simulink model "Task4_4"  (R2020b)
settings: Solver=ode23t  StartTime=0.0  StopTime=300  FixedStep=1e-4  RelTol=1e-3
values from neighbouring files (symbols this model uses):
  Cp_opt = lambda_opt * Ct_opt    (= 0.4375971)    [Code2021_Jo_Saleh.m]    (also in ExeRet21.m.m)
  Ct = c0 + c1.*lambda + c2*lambda.^2    [Code2021_Jo_Saleh.m]    (also in ExeRet21.m.m)
  i_sd_mat = zeros(1, length(Te))    [Code2021_Jo_Saleh.m]    (also in ExeRet21.m.m)
  i_sq_mat = zeros(1, length(Te))    [Code2021_Jo_Saleh.m]    (also in ExeRet21.m.m)
  J = H * 2 * Sb / wm^2    (= 9574851.8542)    [Code2021_Jo_Saleh.m]    (also in ExeRet21.m.m)
  K = p * tau_z / (tau_pl * 2*we * tau_w)    (= -13.4008504823)    [Code2021_Jo_Saleh.m]    (also in ExeRet21.m.m)
  Kd_i = Rs * Kd_p / Lsd    (= -20)    [Code2021_Jo_Saleh.m]    (also in ExeRet21.m.m)
  Kd_p = - Lsd / tau_i    (= -2)    [Code2021_Jo_Saleh.m]    (also in ExeRet21.m.m)
  Kq_i = Rs * Kq_p / Lsq    (= -20)    [Code2021_Jo_Saleh.m]    (also in ExeRet21.m.m)
  Kq_p = - Lsq / tau_i    (= -2.66666666667)    [Code2021_Jo_Saleh.m]    (also in ExeRet21.m.m)
  lambda_opt = 6.7    [Code2021_Jo_Saleh.m]    (also in ExeRet21.m.m)
  Lsd = 6e-3    (= 0.006)    [Code2021_Jo_Saleh.m]    (also in ExeRet21.m.m)
  Lsq = 8e-3    (= 0.008)    [Code2021_Jo_Saleh.m]    (also in ExeRet21.m.m)
  p = 180    [Code2021_Jo_Saleh.m]    (also in ExeRet21.m.m)
  Phi_m = 17.3    [Code2021_Jo_Saleh.m]    (also in ExeRet21.m.m)
  r = 50    [Code2021_Jo_Saleh.m]    (also in ExeRet21.m.m)
  rho = 1.225    [Code2021_Jo_Saleh.m]    (also in ExeRet21.m.m)
  Rs = 60e-3    (= 0.06)    [Code2021_Jo_Saleh.m]    (also in ExeRet21.m.m)
  tau_le = tau_w    (= 8.82652066845)    [Code2021_Jo_Saleh.m]    (also in ExeRet21.m.m)
  tau_lg = tau_z    (= -109.330180381)    [Code2021_Jo_Saleh.m]    (also in ExeRet21.m.m)
  Te = 0:1e3:Te_rated    [Code2021_Jo_Saleh.m]    (also in ExeRet21.m.m)
  Te_rated = (Ptur * p) / (2 * we)    (= 1671126.90246)    [Code2021_Jo_Saleh.m]    (also in ExeRet21.m.m)
  Vdc = 6e3    (= 6000)    [Code2021_Jo_Saleh.m]    (also in ExeRet21.m.m)
libraries: pid_lib x2
settings Model: Creator=Tomo  LastModifiedBy=Tomo

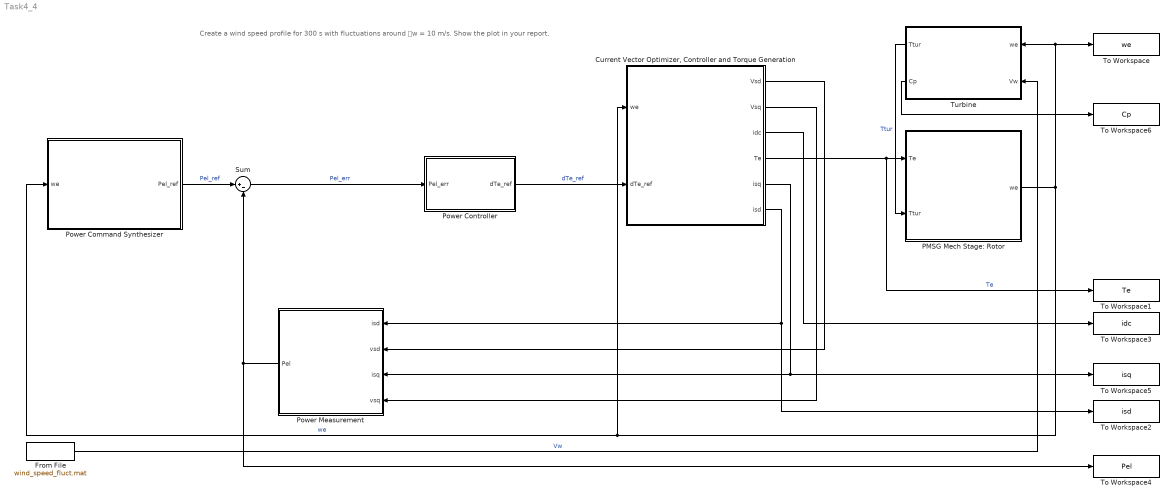
== system Task4_4 ==
  note: Create a wind speed profile for 300 s with fluctuations around 𝑉w = 10 m/s. Show the plot in your report.
  "Current Vector Optimizer, Controller and Torque Generation" : Subsystem
  From File : FromFile  FileName=wind_speed_fluct.mat  SampleTime=0
  PMSG Mech Stage: Rotor : Subsystem
  Power Command Synthesizer : Subsystem
  Power Controller : Subsystem
  Power Measurement : Subsystem
  Sum : Sum  Inputs=|+-
  To Workspace : ToWorkspace  VariableName=we  SampleTime=-1
  To Workspace1 : ToWorkspace  VariableName=Te  SampleTime=-1
  To Workspace2 : ToWorkspace  VariableName=isd  SampleTime=-1
  To Workspace3 : ToWorkspace  VariableName=idc  SampleTime=-1
  To Workspace4 : ToWorkspace  VariableName=Pel  SampleTime=-1
  To Workspace5 : ToWorkspace  VariableName=isq  SampleTime=-1
  To Workspace6 : ToWorkspace  VariableName=Cp  SampleTime=-1
  Turbine : Subsystem
  wires:
  "Current Vector Optimizer, Controller and Torque Generation"/3(idc) -> To Workspace3/1
  "Current Vector Optimizer, Controller and Torque Generation"/4(Te) -> To Workspace1/1, PMSG Mech Stage: Rotor/1(Te)  "Te"
  Power Measurement/1(Pel) -> Sum/2, To Workspace4/1
  "Current Vector Optimizer, Controller and Torque Generation"/2(Vsq) -> Power Measurement/4(vsq)
  Sum/1 -> Power Controller/1(Pel_err)  "Pel_err"
  From File/1 -> Turbine/2(Vw)  "Vw"
  PMSG Mech Stage: Rotor/1(we) -> "Current Vector Optimizer, Controller and Torque Generation"/1(we), Power Command Synthesizer/1(we), To Workspace/1, Turbine/1(we)  "we"
  "Current Vector Optimizer, Controller and Torque Generation"/6(isd) -> To Workspace2/1, Power Measurement/1(isd)
  Turbine/1(Ttur) -> PMSG Mech Stage: Rotor/2(Ttur)  "Ttur"
  Power Command Synthesizer/1(Pel_ref) -> Sum/1  "Pel_ref"
  "Current Vector Optimizer, Controller and Torque Generation"/5(isq) -> To Workspace5/1, Power Measurement/3(isq)
  Power Controller/1(dTe_ref) -> "Current Vector Optimizer, Controller and Torque Generation"/2(dTe_ref)  "dTe_ref"
  "Current Vector Optimizer, Controller and Torque Generation"/1(Vsd) -> Power Measurement/2(vsd)
  Turbine/2(Cp) -> To Workspace6/1

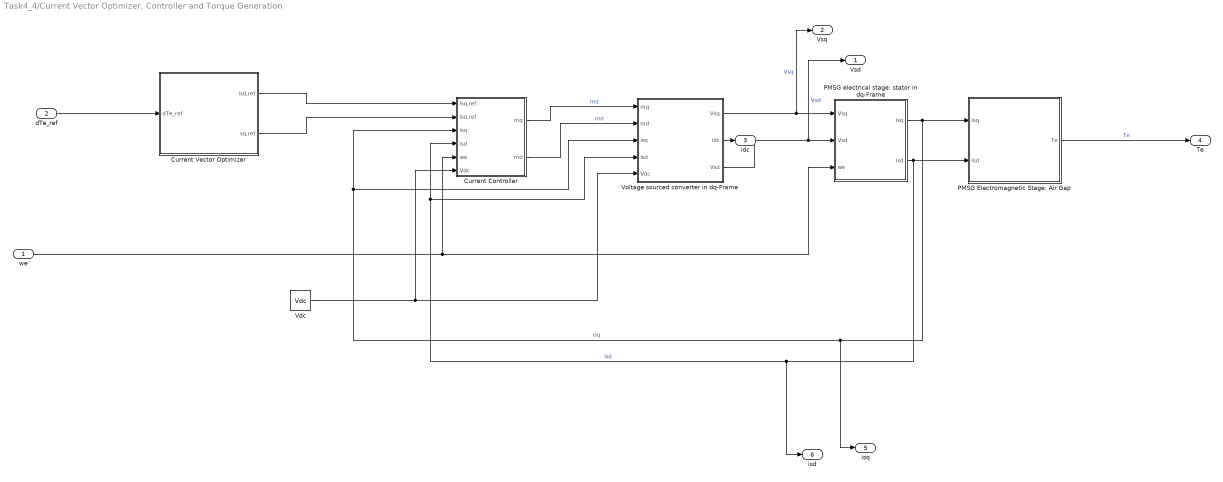
== system Task4_4/Current Vector Optimizer, Controller and Torque Generation ==
  we : Inport
  dTe_ref : Inport  Port=2
  Current Controller : Subsystem
  Current Vector Optimizer : Subsystem
  PMSG Electromagnetic Stage: Air Gap : Subsystem
  PMSG electrical stage: stator in dq-Frame : Subsystem
  Vdc : Constant  Value=Vdc
  Voltage sourced converter in dq-Frame : Subsystem
  Vsd : Outport
  Vsq : Outport  Port=2
  idc : Outport  Port=3
  Te : Outport  Port=4
  isq : Outport  Port=5
  isd : Outport  Port=6
  wires:
  PMSG electrical stage: stator in dq-Frame/1(isq) -> isq/1, Voltage sourced converter in dq-Frame/3(isq), Current Controller/3(isq), PMSG Electromagnetic Stage: Air Gap/1(Isq)  "isq"
  PMSG Electromagnetic Stage: Air Gap/1(Te) -> Te/1  "Te"
  Vdc/1 -> Voltage sourced converter in dq-Frame/5(Vdc), Current Controller/6(Vdc)
  Current Controller/2(md) -> Voltage sourced converter in dq-Frame/2(md)  "md"
  Current Controller/1(mq) -> Voltage sourced converter in dq-Frame/1(mq)  "mq"
  Voltage sourced converter in dq-Frame/1(Vsq) -> Vsq/1, PMSG electrical stage: stator in dq-Frame/1(Vsq)  "Vsq"
  Current Vector Optimizer/2(sq,ref) -> Current Controller/2(isd,ref)
  we/1 -> PMSG electrical stage: stator in dq-Frame/3(we), Current Controller/5(we)
  Voltage sourced converter in dq-Frame/3(Vsd) -> Vsd/1, PMSG electrical stage: stator in dq-Frame/2(Vsd)  "Vsd"
  PMSG electrical stage: stator in dq-Frame/2(isd) -> PMSG Electromagnetic Stage: Air Gap/2(Isd), isd/1, Voltage sourced converter in dq-Frame/4(isd), Current Controller/4(isd)  "isd"
  Current Vector Optimizer/1(isd,ref) -> Current Controller/1(isq,ref)
  Voltage sourced converter in dq-Frame/2(idc) -> idc/1
  dTe_ref/1 -> Current Vector Optimizer/1(dTe_ref)

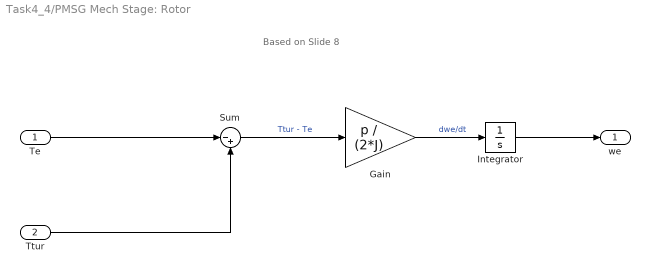
== system Task4_4/PMSG Mech Stage: Rotor ==
  note: Based on Slide 8
  Te : Inport
  Ttur : Inport  Port=2
  Gain : Gain  Gain=p / (2*J)
  Integrator : Integrator  InitialCondition=10
  Sum : Sum  Inputs=|-+
  we : Outport
  wires:
  Gain/1 -> Integrator/1  "dwe/dt"
  Integrator/1 -> we/1
  Sum/1 -> Gain/1  "Ttur - Te"
  Te/1 -> Sum/1
  Ttur/1 -> Sum/2

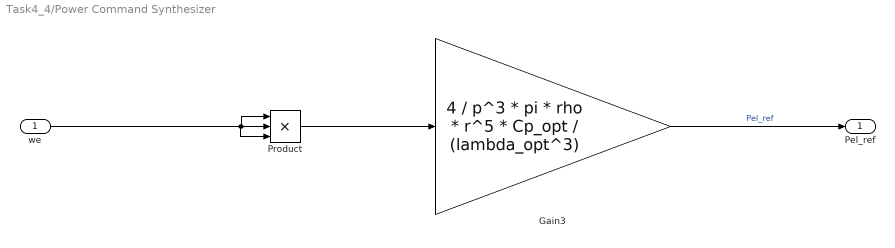
== system Task4_4/Power Command Synthesizer ==
  we : Inport
  Gain3 : Gain  Gain=4 / p^3 * pi * rho * r^5 * Cp_opt / (lambda_opt^3)
  Product : Product  Inputs=3
  Pel_ref : Outport
  wires:
  we/1 -> Product/2, Product/1, Product/3
  Gain3/1 -> Pel_ref/1  "Pel_ref"
  Product/1 -> Gain3/1

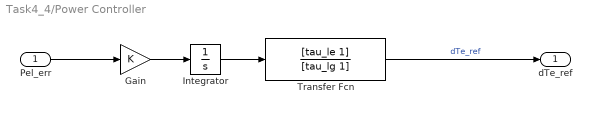
== system Task4_4/Power Controller ==
  Pel_err : Inport
  Gain : Gain  Gain=K
  Integrator : Integrator  InitialCondition=Te_rated
  Transfer Fcn : TransferFcn  Numerator=[tau_le 1]  Denominator=[tau_lg 1]
  dTe_ref : Outport
  wires:
  Transfer Fcn/1 -> dTe_ref/1  "dTe_ref"
  Gain/1 -> Integrator/1
  Integrator/1 -> Transfer Fcn/1
  Pel_err/1 -> Gain/1

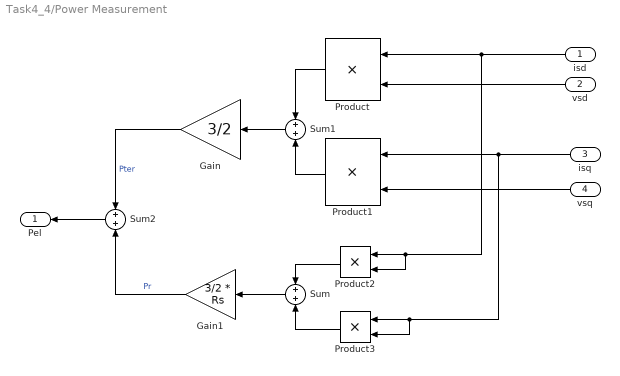
== system Task4_4/Power Measurement ==
  isd : Inport
  vsd : Inport  Port=2
  isq : Inport  Port=3
  vsq : Inport  Port=4
  Gain : Gain  Gain=3/2
  Gain1 : Gain  Gain=3/2 * Rs
  Product{,1..3} (4 alike) : Product
  Sum : Sum  Inputs=+|+
  Sum1 : Sum  Inputs=+|+
  Sum2 : Sum  Inputs=+|+
  Pel : Outport
  wires:
  Product/1 -> Sum1/1
  Sum1/1 -> Gain/1
  vsd/1 -> Product/2
  vsq/1 -> Product1/2
  Gain/1 -> Sum2/1  "Pter"
  isd/1 -> Product2/2, Product2/1, Product/1
  Product1/1 -> Sum1/2
  isq/1 -> Product3/2, Product3/1, Product1/1
  Sum/1 -> Gain1/1
  Product2/1 -> Sum/1
  Product3/1 -> Sum/2
  Gain1/1 -> Sum2/2  "Pr"
  Sum2/1 -> Pel/1

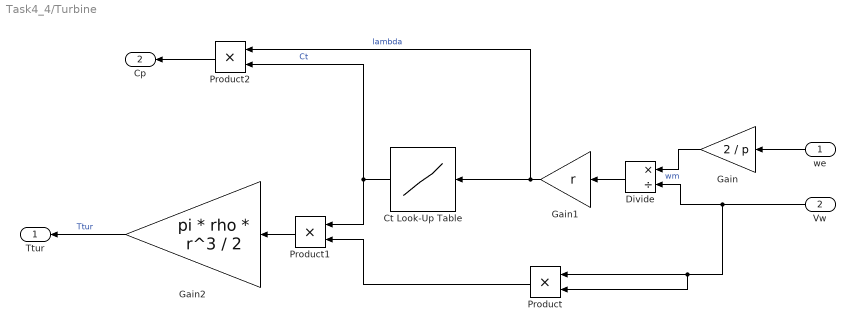
== system Task4_4/Turbine ==
  we : Inport
  Vw : Inport  Port=2
  Ct Look-Up Table : Lookup_n-D  NumberOfTableDimensions=1  BreakpointsForDimension1=[0:1e-2:20]  Table=Ct  InternalRulePriority=Speed  RndMeth=Simplest  InputSameDT=on
  Divide : Product  Inputs=*/
  Gain : Gain  Gain=2 / p
  Gain1 : Gain  Gain=r
  Gain2 : Gain  Gain=pi * rho * r^3 / 2
  Product : Product
  Product1 : Product
  Product2 : Product
  Ttur : Outport
  Cp : Outport  Port=2
  wires:
  we/1 -> Gain/1
  Gain2/1 -> Ttur/1  "Ttur"
  Ct Look-Up Table/1 -> Product1/1, Product2/2  "Ct"
  Gain/1 -> Divide/1  "wm"
  Gain1/1 -> Product2/1, Ct Look-Up Table/1  "lambda"
  Vw/1 -> Product/2, Product/1, Divide/2
  Divide/1 -> Gain1/1
  Product/1 -> Product1/2
  Product1/1 -> Gain2/1
  Product2/1 -> Cp/1

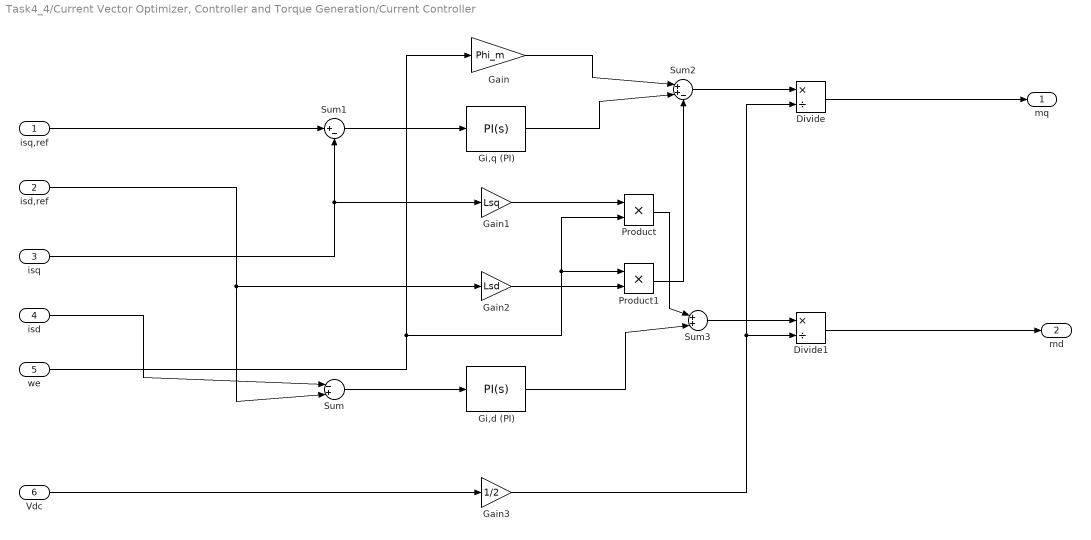
== system Task4_4/Current Vector Optimizer, Controller and Torque Generation/Current Controller ==
  isq,ref : Inport
  isd,ref : Inport  Port=2
  isq : Inport  Port=3
  isd : Inport  Port=4
  we : Inport  Port=5
  Vdc : Inport  Port=6
  Divide : Product  Inputs=*/
  Divide1 : Product  Inputs=*/
  Gain : Gain  Gain=Phi_m
  Gain1 : Gain  Gain=Lsq
  Gain2 : Gain  Gain=Lsd
  Gain3 : Gain  Gain=1/2
  Gi,d (PI) : pid_lib/PID Controller  Controller=PI  Form=Parallel  TimeDomain=Continuous-time  UseExternalTs=off  SampleTime=-1  IntegratorMethod=Forward Euler  FilterMethod=Forward Euler  ControllerParametersSource=internal  P=Kd_p  I=Kd_i  D=0  UseFilter=on  N=100  TunerSelectOption=Transfer Function Based (PID Tuner App)  InitialConditionSource=internal  InitialConditionForIntegrator=0  InitialConditionForFilter=0  DifferentiatorICPrevScaledInput=0  ExternalReset=none  TrackingMode=off  Kt=1  LimitOutput=off  SatLimitsSource=internal  UpperSaturationLimit=inf  LowerSaturationLimit=-inf  LinearizeAsGain=on  AntiWindupMode=none  Kb=1  POutMin=[]  POutMax=[]  IOutMin=[]  IOutMax=[]  DOutMin=[]  DOutMax=[]  NOutMin=[]  NOutMax=[]  SumOutMin=[]  SumOutMax=[]  SaturationOutMin=[]  SaturationOutMax=[]  PParamMin=[]  PParamMax=[]  IParamMin=[]  IParamMax=[]  DParamMin=[]  DParamMax=[]  NParamMin=[]  NParamMax=[]  KbParamMin=[]  KbParamMax=[]  KtParamMin=[]  KtParamMax=[]  KbOutMin=[]  KbOutMax=[]  KtOutMin=[]  KtOutMax=[]  IntegratorOutMin=[]  IntegratorOutMax=[]  FilterOutMin=[]  FilterOutMax=[]  SumI1OutMin=[]  SumI1OutMax=[]  SumI2OutMin=[]  SumI2OutMax=[]  SumI3OutMin=[]  SumI3OutMax=[]  SumI4OutMin=[]  SumI4OutMax=[]  SumDOutMin=[]  SumDOutMax=[]  DifferentiatorOutMin=[]  DifferentiatorOutMax=[]  FilterDiffOutCoefMin=[]  FilterDiffOutCoefMax=[]  ReciprocalOutMin=[]  ReciprocalOutMax=[]  SumDenOutMin=[]  SumDenOutMax=[]  SumNumOutMin=[]  SumNumOutMax=[]  DivideOutMin=[]  DivideOutMax=[]  UdiffTsProdOutMin=[]  UdiffTsProdOutMax=[]  NTsProdOutMin=[]  NTsProdOutMax=[]  UintegralTsProdOutMin=[]  UintegralTsProdOutMax=[]  UngainTsProdOutMin=[]  UngainTsProdOutMax=[]  IntegratorContinuousStateAttributes=''  IntegratorStateMustResolveToSignalObject=off  IntegratorRTWStateStorageClass=Auto  FilterContinuousStateAttributes=''  FilterStateMustResolveToSignalObject=off  FilterRTWStateStorageClass=Auto  ParallelPVariant=InternalParameters  IdealPVariant=Disabled  IVariant=InternalParameters  DVariant=Disabled  IntegratorVariant=Continuous  SatVariant=Disabled  AWVariant=Passthrough  PCopyVariant=Disabled  TRVariant=Disabled  FdbkBlocksVariant=Forward  IdealPFdbkVariant=Disabled  SatFdbkVariant=Disabled  DerivativeFilterVariant=Disabled  NVariant=Disabled  NCopyVariant=Disabled_SignalSpec  FilterICVariant=Disabled  IntegratorICVariant=InternalICs  ExternalResetVariant=Disabled  TRSumVariant=Passthrough  SumFdbkVariant=Disabled  SumVariant=Sum_PI  TsampFilterVariant=InternalTs  TsampNgainVariant=Passthrough  TsampIntegralVariant=Passthrough  ExternalSaturationOutDataTypeStr=Inherit: Same as second input
  Gi,q (PI) : pid_lib/PID Controller  Controller=PI  Form=Parallel  TimeDomain=Continuous-time  UseExternalTs=off  SampleTime=-1  IntegratorMethod=Forward Euler  FilterMethod=Forward Euler  ControllerParametersSource=internal  P=Kq_p  I=Kq_i  D=0  UseFilter=on  N=100  TunerSelectOption=Transfer Function Based (PID Tuner App)  InitialConditionSource=internal  InitialConditionForIntegrator=0  InitialConditionForFilter=0  DifferentiatorICPrevScaledInput=0  ExternalReset=none  TrackingMode=off  Kt=1  LimitOutput=off  SatLimitsSource=internal  UpperSaturationLimit=inf  LowerSaturationLimit=-inf  LinearizeAsGain=on  AntiWindupMode=none  Kb=1  POutMin=[]  POutMax=[]  IOutMin=[]  IOutMax=[]  DOutMin=[]  DOutMax=[]  NOutMin=[]  NOutMax=[]  SumOutMin=[]  SumOutMax=[]  SaturationOutMin=[]  SaturationOutMax=[]  PParamMin=[]  PParamMax=[]  IParamMin=[]  IParamMax=[]  DParamMin=[]  DParamMax=[]  NParamMin=[]  NParamMax=[]  KbParamMin=[]  KbParamMax=[]  KtParamMin=[]  KtParamMax=[]  KbOutMin=[]  KbOutMax=[]  KtOutMin=[]  KtOutMax=[]  IntegratorOutMin=[]  IntegratorOutMax=[]  FilterOutMin=[]  FilterOutMax=[]  SumI1OutMin=[]  SumI1OutMax=[]  SumI2OutMin=[]  SumI2OutMax=[]  SumI3OutMin=[]  SumI3OutMax=[]  SumI4OutMin=[]  SumI4OutMax=[]  SumDOutMin=[]  SumDOutMax=[]  DifferentiatorOutMin=[]  DifferentiatorOutMax=[]  FilterDiffOutCoefMin=[]  FilterDiffOutCoefMax=[]  ReciprocalOutMin=[]  ReciprocalOutMax=[]  SumDenOutMin=[]  SumDenOutMax=[]  SumNumOutMin=[]  SumNumOutMax=[]  DivideOutMin=[]  DivideOutMax=[]  UdiffTsProdOutMin=[]  UdiffTsProdOutMax=[]  NTsProdOutMin=[]  NTsProdOutMax=[]  UintegralTsProdOutMin=[]  UintegralTsProdOutMax=[]  UngainTsProdOutMin=[]  UngainTsProdOutMax=[]  IntegratorContinuousStateAttributes=''  IntegratorStateMustResolveToSignalObject=off  IntegratorRTWStateStorageClass=Auto  FilterContinuousStateAttributes=''  FilterStateMustResolveToSignalObject=off  FilterRTWStateStorageClass=Auto  ParallelPVariant=InternalParameters  IdealPVariant=Disabled  IVariant=InternalParameters  DVariant=Disabled  IntegratorVariant=Continuous  SatVariant=Disabled  AWVariant=Passthrough  PCopyVariant=Disabled  TRVariant=Disabled  FdbkBlocksVariant=Forward  IdealPFdbkVariant=Disabled  SatFdbkVariant=Disabled  DerivativeFilterVariant=Disabled  NVariant=Disabled  NCopyVariant=Disabled_SignalSpec  FilterICVariant=Disabled  IntegratorICVariant=InternalICs  ExternalResetVariant=Disabled  TRSumVariant=Passthrough  SumFdbkVariant=Disabled  SumVariant=Sum_PI  TsampFilterVariant=InternalTs  TsampNgainVariant=Passthrough  TsampIntegralVariant=Passthrough  ExternalSaturationOutDataTypeStr=Inherit: Same as second input
  Product : Product
  Product1 : Product
  Sum : Sum  Inputs=|-+|
  Sum1 : Sum  Inputs=|+-
  Sum2 : Sum  Inputs=|++-
  Sum3 : Sum  Inputs=|++|
  mq : Outport
  md : Outport  Port=2
  wires:
  Gain3/1 -> Divide/2, Divide1/2
  we/1 -> Gain/1, Product/2, Product1/1
  Sum/1 -> Gi,d (PI)/1
  Vdc/1 -> Gain3/1
  Sum3/1 -> Divide1/1
  isq/1 -> Gain1/1, Sum1/2
  Sum1/1 -> Gi,q (PI)/1
  Gain/1 -> Sum2/1
  Gain2/1 -> Product1/2
  isd,ref/1 -> Sum/2, Gain2/1
  Sum2/1 -> Divide/1
  Gi,d (PI)/1 -> Sum3/2
  Product/1 -> Sum3/1
  Product1/1 -> Sum2/3
  Gain1/1 -> Product/1
  isq,ref/1 -> Sum1/1
  Gi,q (PI)/1 -> Sum2/2
  Divide/1 -> mq/1
  isd/1 -> Sum/1
  Divide1/1 -> md/1

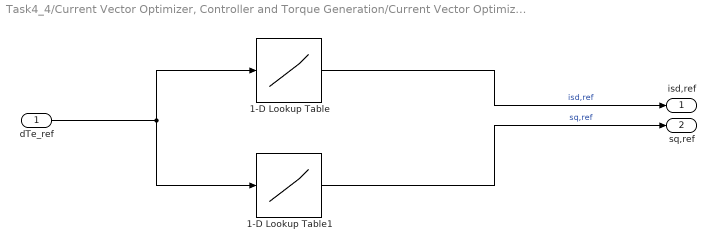
== system Task4_4/Current Vector Optimizer, Controller and Torque Generation/Current Vector Optimizer ==
  dTe_ref : Inport
  1-D Lookup Table : Lookup_n-D  NumberOfTableDimensions=1  BreakpointsForDimension1=Te  Table=i_sd_mat  InternalRulePriority=Speed  RndMeth=Simplest  InputSameDT=on
  1-D Lookup Table1 : Lookup_n-D  NumberOfTableDimensions=1  BreakpointsForDimension1=Te  Table=i_sq_mat  InternalRulePriority=Speed  RndMeth=Simplest  InputSameDT=on
  isd,ref : Outport
  sq,ref : Outport  Port=2
  wires:
  dTe_ref/1 -> 1-D Lookup Table/1, 1-D Lookup Table1/1
  1-D Lookup Table/1 -> isd,ref/1  "isd,ref"
  1-D Lookup Table1/1 -> sq,ref/1  "sq,ref"

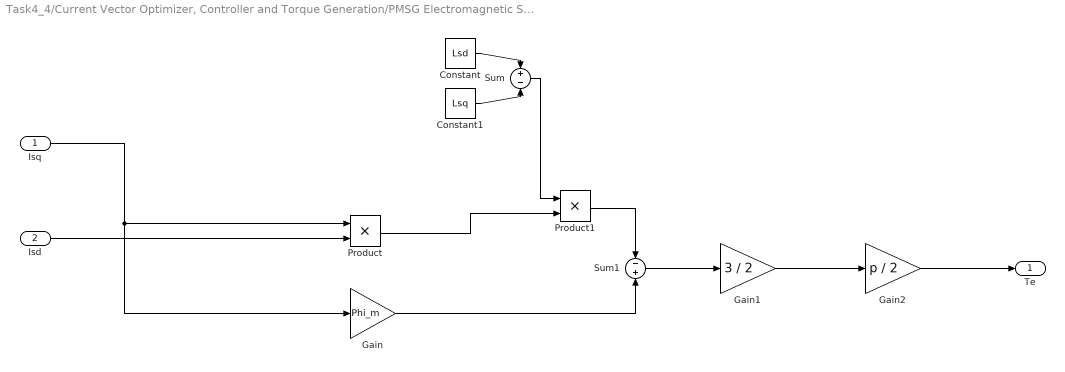
== system Task4_4/Current Vector Optimizer, Controller and Torque Generation/PMSG Electromagnetic Stage: Air Gap ==
  Isq : Inport
  Isd : Inport  Port=2
  Constant : Constant  Value=Lsd
  Constant1 : Constant  Value=Lsq
  Gain : Gain  Gain=Phi_m
  Gain1 : Gain  Gain=3 / 2
  Gain2 : Gain  Gain=p / 2
  Product : Product
  Product1 : Product
  Sum : Sum  Inputs=+-
  Sum1 : Sum  Inputs=-+
  Te : Outport
  wires:
  Isq/1 -> Gain/1, Product/1
  Product/1 -> Product1/2
  Sum1/1 -> Gain1/1
  Sum/1 -> Product1/1
  Isd/1 -> Product/2
  Constant1/1 -> Sum/2
  Product1/1 -> Sum1/1
  Gain/1 -> Sum1/2
  Constant/1 -> Sum/1
  Gain2/1 -> Te/1
  Gain1/1 -> Gain2/1

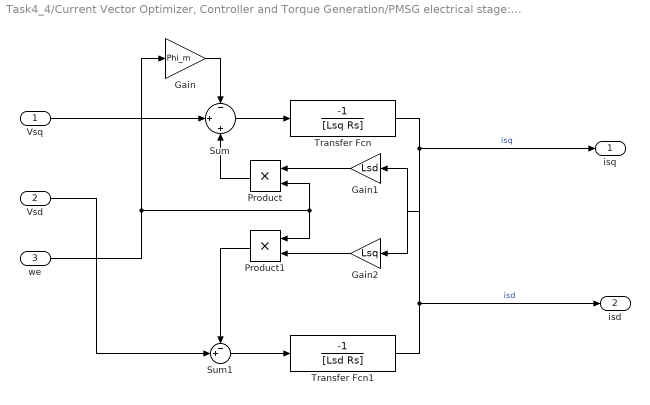
== system Task4_4/Current Vector Optimizer, Controller and Torque Generation/PMSG electrical stage: stator in dq-Frame ==
  Vsq : Inport
  Vsd : Inport  Port=2
  we : Inport  Port=3
  Gain : Gain  Gain=Phi_m
  Gain1 : Gain  Gain=Lsd
  Gain2 : Gain  Gain=Lsq
  Product : Product
  Product1 : Product
  Sum : Sum  Inputs=-|+|+
  Sum1 : Sum  Inputs=-+|
  Transfer Fcn : TransferFcn  Numerator=[-1]  Denominator=[Lsq Rs]
  Transfer Fcn1 : TransferFcn  Numerator=[-1]  Denominator=[Lsd Rs]
  isq : Outport
  isd : Outport  Port=2
  wires:
  Sum/1 -> Transfer Fcn/1
  Product/1 -> Sum/3
  Gain/1 -> Sum/1
  we/1 -> Gain/1, Product/2, Product1/1
  Transfer Fcn1/1 -> Gain1/1, isd/1  "isd"
  Vsq/1 -> Sum/2
  Transfer Fcn/1 -> Gain2/1, isq/1  "isq"
  Product1/1 -> Sum1/1
  Sum1/1 -> Transfer Fcn1/1
  Vsd/1 -> Sum1/2
  Gain1/1 -> Product/1
  Gain2/1 -> Product1/2

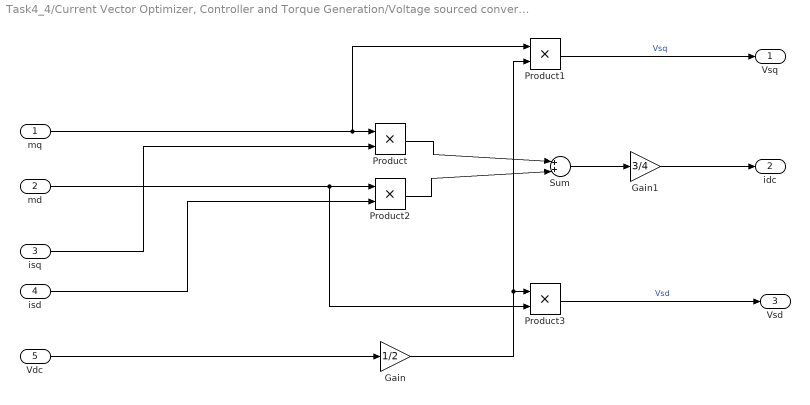
== system Task4_4/Current Vector Optimizer, Controller and Torque Generation/Voltage sourced converter in dq-Frame ==
  mq : Inport
  md : Inport  Port=2
  isq : Inport  Port=3
  isd : Inport  Port=4
  Vdc : Inport  Port=5
  Gain : Gain  Gain=1/2
  Gain1 : Gain  Gain=3/4
  Product{,1..3} (4 alike) : Product
  Sum : Sum  Inputs=|++|
  Vsq : Outport
  idc : Outport  Port=2
  Vsd : Outport  Port=3
  wires:
  Product2/1 -> Sum/2
  mq/1 -> Product1/1, Product/1
  Gain/1 -> Product1/2, Product3/1
  isd/1 -> Product2/2
  Vdc/1 -> Gain/1
  md/1 -> Product3/2, Product2/1
  Product3/1 -> Vsd/1  "Vsd"
  Product1/1 -> Vsq/1  "Vsq"
  Sum/1 -> Gain1/1
  isq/1 -> Product/2
  Product/1 -> Sum/1
  Gain1/1 -> idc/1
